simulink model "Blending_Tank_Transfer_Functions"  (R2015b)
settings: Solver=VariableStepAuto  StartTime=0.0  StopTime=20  RelTol=1e-3
settings Model: Creator=Emsnuelly  LastModifiedBy=Emsnuelly

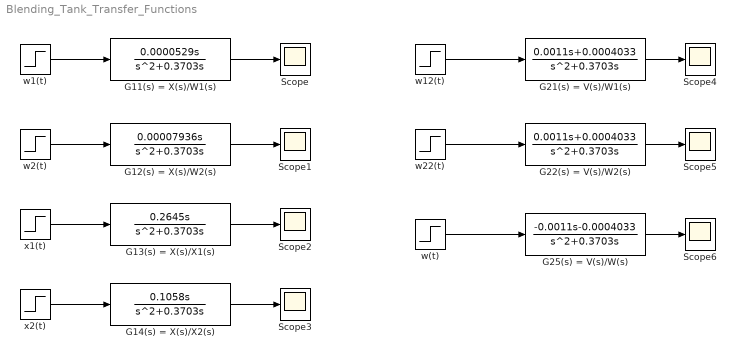
== system Blending_Tank_Transfer_Functions ==
  G11(s) = X(s)/W1(s) : TransferFcn  Numerator=[0.0000529 0]  Denominator=[1 0.3703 0]
  G12(s) = X(s)/W2(s) : TransferFcn  Numerator=[0.00007936 0]  Denominator=[1 0.3703 0]
  G13(s) = X(s)/X1(s) : TransferFcn  Numerator=[0.2645 0]  Denominator=[1 0.3703 0]
  G14(s) = X(s)/X2(s) : TransferFcn  Numerator=[0.1058 0]  Denominator=[1 0.3703 0]
  G21(s) = V(s)/W1(s) : TransferFcn  Numerator=[0.0011 0.0004033]  Denominator=[1 0.3703 0]
  G22(s) = V(s)/W2(s) : TransferFcn  Numerator=[0.0011 0.0004033]  Denominator=[1 0.3703 0]
  G25(s) = V(s)/W(s) : TransferFcn  Numerator=[-0.0011 -0.0004033]  Denominator=[1 0.3703 0]
  Scope{,1..6} (7 alike) : Scope
  w(t) : Step  After=650  SampleTime=0
  w1(t) : Step  After=500  SampleTime=0
  w12(t) : Step  After=500  SampleTime=0
  w2(t) : Step  After=200  SampleTime=0
  w22(t) : Step  After=200  SampleTime=0
  x1(t) : Step  After=0.4  SampleTime=0
  x2(t) : Step  After=0.75  SampleTime=0
  wires:
  x2(t)/1 -> G14(s) = X(s)/X2(s)/1
  x1(t)/1 -> G13(s) = X(s)/X1(s)/1
  w2(t)/1 -> G12(s) = X(s)/W2(s)/1
  w1(t)/1 -> G11(s) = X(s)/W1(s)/1
  w12(t)/1 -> G21(s) = V(s)/W1(s)/1
  w22(t)/1 -> G22(s) = V(s)/W2(s)/1
  w(t)/1 -> G25(s) = V(s)/W(s)/1
  G11(s) = X(s)/W1(s)/1 -> Scope/1
  G12(s) = X(s)/W2(s)/1 -> Scope1/1
  G13(s) = X(s)/X1(s)/1 -> Scope2/1
  G14(s) = X(s)/X2(s)/1 -> Scope3/1
  G21(s) = V(s)/W1(s)/1 -> Scope4/1
  G22(s) = V(s)/W2(s)/1 -> Scope5/1
  G25(s) = V(s)/W(s)/1 -> Scope6/1
